simulink model "Adams_HW_Dynamic"  (R2023b)
settings: Solver=VariableStepAuto  StartTime=0.0  StopTime=10.0  RelTol=1e-3
values from neighbouring files (symbols this model uses):
  J1 = (1/3)*m1*L1^2    [Adams_HW1.m]
  J2 = (1/12)*m2*L2^2    [Adams_HW1.m]
  J3 = (1/3)*m3*L3^2    [Adams_HW1.m]
  L1 = x(1)    [Adams_HW1.m]    (also in Adams_HW_DrawGIF.m = current_x(1); Adams_HW_DrawGIF_Y.m = current_x(1))
  L2 = x(2)    [Adams_HW1.m]    (also in Adams_HW_DrawGIF.m = current_x(2); Adams_HW_DrawGIF_Y.m = current_x(2))
  L3 = x(3)    [Adams_HW1.m]    (also in Adams_HW_DrawGIF.m = current_x(3); Adams_HW_DrawGIF_Y.m = current_x(3))
  L4 = x(4)    [Adams_HW1.m]    (also in Adams_HW_DrawGIF.m = current_x(4); Adams_HW_DrawGIF_Y.m = current_x(4))
  M = -5    [Adams_HW1.m]
  m1 = 5    [Adams_HW1.m]
  m2 = 5    [Adams_HW1.m]
  m3 = 5    [Adams_HW1.m]
  Q1 = x(5)    [Adams_HW1.m]    (also in Adams_HW_DrawGIF.m = current_x(5); Adams_HW_DrawGIF_Y.m = current_x(5))
  Q2 = Inition(1)    [Adams_HW1.m]
  Q3 = x(11)    [Adams_HW1.m]    (also in Adams_HW_DrawGIF.m = current_x(11); Adams_HW_DrawGIF_Y.m = current_x(7))
settings Model: Creator=Akko  LastModifiedBy=Akko

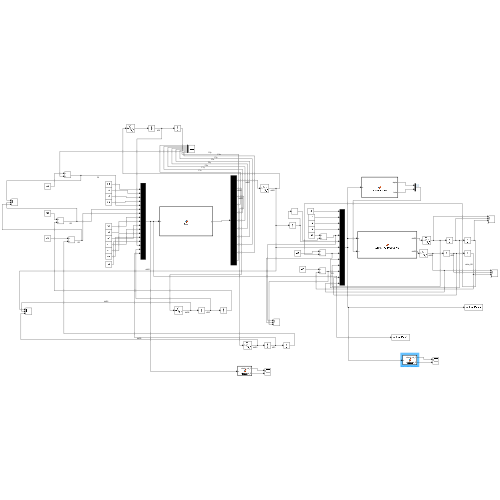
[thumbnail: Simulink's stored preview of the top-level diagram]
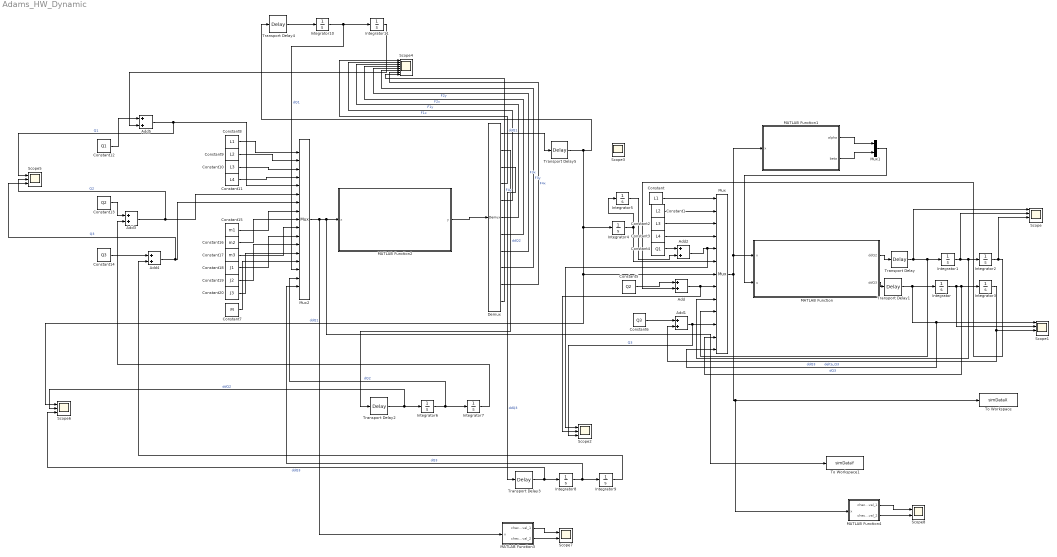
== system Adams_HW_Dynamic ==
  Add{,1..5} (6 alike) : Sum
  Constant : Constant  Value=L1
  Constant1 : Constant  Value=L2
  Constant10 : Constant  Value=L3
  Constant11 : Constant  Value=L4
  Constant12 : Constant  Value=Q1
  Constant13 : Constant  Value=Q2
  Constant14 : Constant  Value=Q3
  Constant15 : Constant  Value=m1
  Constant16 : Constant  Value=m2
  Constant17 : Constant  Value=m3
  Constant18 : Constant  Value=J1
  Constant19 : Constant  Value=J2
  Constant2 : Constant  Value=L3
  Constant20 : Constant  Value=J3
  Constant3 : Constant  Value=L4
  Constant4 : Constant  Value=Q1
  Constant5 : Constant  Value=Q2
  Constant6 : Constant  Value=Q3
  Constant7 : Constant  Value=M
  Constant8 : Constant  Value=L1
  Constant9 : Constant  Value=L2
  Demux : Demux  Outputs=11
  Integrator{,1..11} (12 alike) : Integrator
  MATLAB Function : MATLAB Function  TreatAsAtomicUnit=on
  MATLAB Function1 : MATLAB Function  TreatAsAtomicUnit=on
  MATLAB Function2 : MATLAB Function  TreatAsAtomicUnit=on
  MATLAB Function3 : MATLAB Function  TreatAsAtomicUnit=on
  MATLAB Function4 : MATLAB Function  TreatAsAtomicUnit=on
  Mux : Mux  Inputs=13
  Mux1 : Mux  Inputs=2
  Mux2 : Mux  Inputs=17
  Scope : Scope  NumInputPorts=4
  Scope1 : Scope  NumInputPorts=4
  Scope2 : Scope  NumInputPorts=3
  Scope4 : Scope  NumInputPorts=8
  Scope5 : Scope  NumInputPorts=3
  Scope6 : Scope  NumInputPorts=3
  Scope7 : Scope  NumInputPorts=2
  Scope8 : Scope  NumInputPorts=2
  To Workspace : ToWorkspace  VariableName=simDataX  SampleTime=-1
  To Workspace1 : ToWorkspace  VariableName=simDataY  SampleTime=-1
  Transport Delay{,1..5} (6 alike) : TransportDelay  DelayTime=1e-4
  Scope3 : Scope
  wires:
  Mux/1 -> MATLAB Function1/1("x "), MATLAB Function/1(x), MATLAB Function4/1(x), To Workspace/1
  Constant/1 -> Mux/1
  Constant1/1 -> Mux/2
  Constant2/1 -> Mux/3
  Constant3/1 -> Mux/4
  MATLAB Function/2(ddQ3) -> Transport Delay1/1
  MATLAB Function/1(ddQ2) -> Transport Delay/1
  Transport Delay1/1 -> Mux/13, Scope1/1, Integrator/1  "ddQ3"
  Transport Delay/1 -> Scope/1, Mux/10, Integrator1/1
  Integrator1/1 -> Scope/2, Mux/9, Integrator2/1
  Integrator/1 -> Scope1/2, Mux/12, Integrator3/1  "dQ3"
  Integrator2/1 -> Scope/3, Add/2
  Constant5/1 -> Add/1
  Add/1 -> Scope2/2, Mux/8
  Add1/1 -> Mux/11, Scope2/3  "Q3"
  Constant6/1 -> Add1/1
  Integrator3/1 -> Scope1/3, Add1/2  "delta_Q3"
  Demux/1 -> Transport Delay5/1  "ddQ1"
  Integrator4/1 -> Integrator5/1, Mux/6
  Add2/1 -> Scope2/1, Mux/5
  Constant4/1 -> Add2/1
  Integrator5/1 -> Add2/2
  MATLAB Function1/1(alpha) -> Mux1/1
  MATLAB Function1/2(beta) -> Mux1/2
  Mux1/1 -> MATLAB Function/2(u)
  Mux2/1 -> MATLAB Function3/1(x), To Workspace1/1, MATLAB Function2/1(x)
  MATLAB Function2/1(y) -> Demux/1
  Constant8/1 -> Mux2/1
  Constant9/1 -> Mux2/2
  Constant10/1 -> Mux2/3
  Constant11/1 -> Mux2/4
  Constant12/1 -> Add5/1
  Constant14/1 -> Add4/1
  Constant16/1 -> Mux2/9
  Constant15/1 -> Mux2/8
  Constant17/1 -> Mux2/10
  Constant18/1 -> Mux2/11
  Constant19/1 -> Mux2/12
  Constant20/1 -> Mux2/13
  Demux/2 -> Transport Delay2/1  "ddQ2"
  Demux/3 -> Transport Delay3/1  "ddQ3"
  Demux/4 -> Scope4/1  "F1x"
  Demux/5 -> Scope4/2  "F1y"
  Demux/6 -> Scope4/3  "F2x"
  Demux/7 -> Scope4/4  "F2y"
  Demux/8 -> Scope4/5  "F3x"
  Demux/9 -> Scope4/6  "F3y"
  Demux/10 -> Scope4/7  "F4x"
  Demux/11 -> Scope4/8  "F4y"
  Constant7/1 -> Mux2/14
  Transport Delay2/1 -> Scope6/2, Integrator6/1  "ddQ2"
  Integrator6/1 -> Mux2/16, Integrator7/1  "dQ2"
  Integrator8/1 -> Mux2/17, Integrator9/1  "dQ3"
  Transport Delay3/1 -> Scope6/3, Integrator8/1  "ddQ3"
  Integrator7/1 -> Add3/2
  Constant13/1 -> Add3/1
  Add3/1 -> Scope5/2, Mux2/6  "Q2"
  Integrator9/1 -> Add4/2
  Add4/1 -> Scope5/3, Mux2/7  "Q3"
  Add5/1 -> Scope5/1, Mux2/5  "Q1"
  Transport Delay4/1 -> Integrator10/1
  Integrator10/1 -> Mux2/15, Integrator11/1  "dQ1"
  Integrator11/1 -> Add5/2
  Transport Delay5/1 -> Transport Delay4/1, Scope6/1, Mux/7, Integrator4/1  "ddQ1"
  MATLAB Function3/1(check_val_1) -> Scope7/1
  MATLAB Function3/2(check_val_2) -> Scope7/2
  MATLAB Function4/2(check_val_2) -> Scope8/2
  MATLAB Function4/1(check_val_1) -> Scope8/1

== matlab function Adams_HW_Dynamic/MATLAB Function ==
  data: x input; ddQ2 output; ddQ3 output; u input
function [ddQ2,ddQ3]=Adams_HW_Dynamic_Cal(x,u)
L1=x(1);L2=x(2);L3=x(3);L4=x(4);
Q1=x(5);dQ1=x(6);ddQ1=x(7);
Q2=x(8);dQ2=x(9);ddQ2=x(10);
Q3=x(11);dQ3=x(12);ddQ3=x(13);
alpha=u(1);beta=u(2);


%BSM法相关定义
%Phi为位置约束列向量
Phi=[ L1*cos(Q1) + L2*cos(Q2) - L3*cos(Q3) - L4;
    L1*sin(Q1) + L2*sin(Q2) - L3*sin(Q3)];

%dot_Phi为速度约束列向量
Jacob=[-L1*sin(Q1),-(L2)*sin(Q2),L3*sin(Q3);
        L1*cos(Q1),(L2)*cos(Q2),-L3*cos(Q3);
];%Q1、Q2、Q3

Phi_t=zeros(2,1);
dot_Phi=Jacob*[dQ1;dQ2;dQ3]+Phi_t;



A_1=[L2*cos(Q2), - L3*cos(Q3);
     L2*sin(Q2) ,- L3*sin(Q3)]*[dQ2^2;dQ3^2];


A_2=[-L2*sin(Q2),  L3*sin(Q3);
      L2*cos(Q2), -L3*cos(Q3)];%*[ddQ2;ddQ3]


b_1=[ L1*sin(Q1); 
     -L1*cos(Q1)]*ddQ1;
b_2=[L1*cos(Q1);L1*sin(Q1)]*((dQ1)^2);

b=((b_1+b_2)-A_1)-(2*alpha*dot_Phi+(beta^2)*Phi);

if abs(det(A_2)) < 1e-6
    % 如果矩阵接近奇异，使用伪逆 (pinv) 或者输出 0 防止报错
    y = pinv(A_2) * b; 
else
    y = A_2\b;
end

ddQ2=y(1);
ddQ3=y(2);
end

== matlab function Adams_HW_Dynamic/MATLAB Function2 ==
  data: x input; y output
function y = force(x)
L1=x(1);L2=x(2);L3=x(3);L4=x(4);
Q1=x(5);
Q2=x(6);
Q3=x(7);
m1=x(8);m2=x(9);m3=x(10);JR1=x(11);J2=x(12);J3=x(13);
M=x(14);dQ1=x(15);dQ2=x(16);dQ3=x(17);


A = zeros(11, 11);
b = zeros(11, 1);

% 预计算三角函数以提高效率
S1 = sin(Q1); C1 = cos(Q1);
S2 = sin(Q2); C2 = cos(Q2);
S3 = sin(Q3); C3 = cos(Q3);

% --- 第1-2行：运动学加速度约束方程 ---
A(1, 1) = -L1 * S1;  A(1, 2) = -L2 * S2;  A(1, 3) =  L3 * S3;
b(1)    =  L1 * C1 * dQ1^2 + L2 * C2 * dQ2^2 - L3 * C3 * dQ3^2;

A(2, 1) =  L1 * C1;  A(2, 2) =  L2 * C2;  A(2, 3) = -L3 * C3;
b(2)    =  L1 * S1 * dQ1^2 + L2 * S2 * dQ2^2 - L3 * S3 * dQ3^2;

% --- 第3-5行：构件 1 (曲柄) 动力学方程 ---
A(3, 1) = m1 * (L1/2) * C1;   A(3, 4) = 1;  A(3, 6) = -1;
A(4, 1) = m1 * (L1/2) * S1;   A(4, 5) = 1;  A(4, 7) = -1;
A(5, 1) = -JR1;               A(5, 6) = L1 * S1;  A(5, 7) = -L1 * C1;
b(5)    = -M;

% --- 第6-8行：构件 2 (连杆) 动力学方程 ---
A(6, 1) = m2 * L1 * C1;  A(6, 2) = m2 * (L2/2) * C2;  A(6, 6) = -1;  A(6, 8) = -1;
A(7, 1) = m2 * L1 * S1;  A(7, 2) = m2 * (L2/2) * S2;  A(7, 7) = -1;  A(7, 9) = -1;
A(8, 2) = -J2;           A(8, 6) = -(L2/2) * S2;      A(8, 7) = (L2/2) * C2;  
                         A(8, 8) = (L2/2) * S2;       A(8, 9) = -(L2/2) * C2;

% --- 第9-11行：构件 3 (摇杆) 动力学方程 ---
A(9, 3)  = m3 * (L3/2) * C3;  A(9, 8) = -1;  A(9, 10) = -1;
A(10, 3) = m3 * (L3/2) * S3;  A(10, 9) = -1;  A(10, 11) = -1;
A(11, 3) = -J3;               A(11, 8) = L3 * S3;  A(11, 9) = L3 * C3;

% --- 求解未知量向量 x ---
% x = [ddQ1; ddQ2; ddQ3; F1x; F1y; F2x; F2y; F3x; F3y; F4x; F4y]
y = A \ b;
end

== matlab function Adams_HW_Dynamic/MATLAB Function3 ==
  data: x input; check_val_1 output; check_val_2 output
function [check_val_1,check_val_2] = detect(x)
L1=x(1);L2=x(2);L3=x(3);L4=x(4);
Q1=x(5);
Q2=x(6);
Q3=x(7);

check_val_1 = L1*cos(Q1) + L2*cos(Q2) - L3*cos(Q3) - L4;
check_val_2 = L1*sin(Q1) + L2*sin(Q2) - L3*sin(Q3);
end

== matlab function Adams_HW_Dynamic/MATLAB Function4 ==
  data: x input; check_val_1 output; check_val_2 output
function [check_val_1,check_val_2] = detect(x)
L1=x(1);L2=x(2);L3=x(3);L4=x(4);
Q1=x(5);
Q2=x(8);
Q3=x(11);

check_val_1 = L1*cos(Q1) + L2*cos(Q2) - L3*cos(Q3) - L4;
check_val_2 = L1*sin(Q1) + L2*sin(Q2) - L3*sin(Q3);
end

== matlab function Adams_HW_Dynamic/MATLAB Function1 ==
  data: x input size=13; alpha output; beta output
function [alpha,beta] = adaptive_BSM(x)
L1=x(1);L2=x(2);L3=x(3);L4=x(4);
Q1=x(5);dQ1=x(6);ddQ1=x(7);
Q2=x(8);dQ2=x(9);ddQ2=x(10);
Q3=x(11);dQ3=x(12);ddQ3=x(13);

    n = 2; % 默认约束方程个数
%BSM法相关定义
%Phi为位置约束列向量
Phi=[ L1*cos(Q1) + L2*cos(Q2) - L3*cos(Q3) - L4;
    L1*sin(Q1) + L2*sin(Q2) - L3*sin(Q3)];

%dot_Phi为速度约束列向量
Jacob=[-L1*sin(Q1),-(L2)*sin(Q2),L3*sin(Q3);
        L1*cos(Q1),(L2)*cos(Q2),-L3*cos(Q3);
];%Q1、Q2、Q3

Phi_t=zeros(2,1);
dot_Phi=Jacob*[dQ1;dQ2;dQ3]+Phi_t;


% 2. 计算模长，加上 eps 防止 log(0)
norm_Phi = sqrt(Phi'*Phi/n);
norm_dotPhi = sqrt(dot_Phi'*dot_Phi/n);

% 使用 log10 替换 lg，并加入 eps 防止负无穷
err_Phi = log10(norm_Phi +eps); 
err_dotPhi = log10(norm_dotPhi +eps); 

%定义计算误差、乘法函数
err=1;%定步长算法

% 定义分段函数
ec = @(z) (z >= -6) * 10 + (z <= -16) * 0 + ...
          (z > -16 & z < -6) .* (16 + z);

y=@(z) 10*err*ec(z);

%计算算子
alpha=y(err_dotPhi);
beta=y(err_Phi);
%做数据保护
alpha = min(max(alpha,0),100); beta = min(max(beta,0),100);
end
